simulink model "simmechanics_inverted_pendulum_v6"  (Simulink 7.6)
settings: Solver=ode4  StartTime=0.0  StopTime=10  FixedStep=step_v  RelTol=1e-3
undefined symbols (not defined in the file or in its folder): g
libraries: mblibv1 x21
settings Model: Creator=pierobon  LastModifiedBy=panics
settings DebuggingCC: StrictBusMsg=Warning
settings SimMechanicsCC: VisOnUpdateDiagram=on  VisDuringSimulation=on  AutoFitVis=GROWTOFIT  LastVizWinPosition=[776 162 684 558]  CamPosition=[-14.9891;0.0801796;0.800186;]  CamTarget=[0;0.0801796;0.800186;]  CamUpVector=[0;1;0;]  CamHeight=5.2311  VisBackgroundColor=[0.729412;0.831373;0.956863;]  DefaultBodyColor=[1;0;0;]

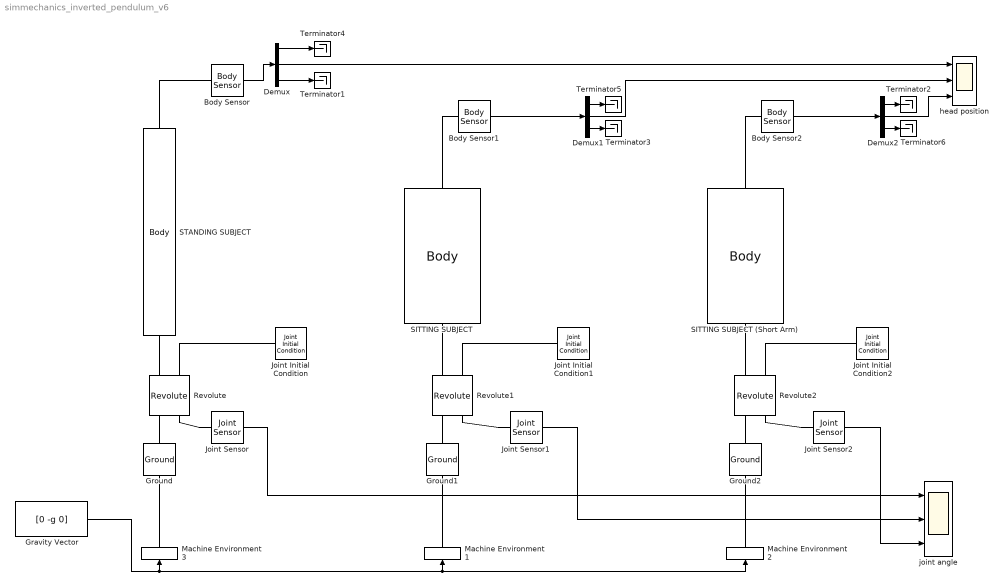
== system simmechanics_inverted_pendulum_v6 ==
  Body Sensor : mblibv1/Sensors &  Actuators/Body Sensor  DialogController=MECH.DynMechDlgSource  SystemSampleTime=-1  UpdateFromCAD=off  PhysicalDomain=Mechanical  PortType=blob  Muxed=off  Pose=off  Angle=on  AngleUnits=deg  ArcVelocity=off  ArcVelocityUnits=deg/s  ArcAcceleration=off  ArcAccelerationUnits=deg/s^2  CoordPosition=on  CoordPositionUnits=in  Velocity=off  VelocityUnits=m/s  Acceleration=off  AccelerationUnits=m/s^2  Quaternion=on  QuaternionDT=off  QuaternionDDT=off  QuaternionUnits=off  OutputVector=[1]  ActiveIO=on  Width=3  DialogClass=MechanicalSensorBlock  ReferenceFrame=Absolute (World)
  Body Sensor1 : mblibv1/Sensors &  Actuators/Body Sensor  DialogController=MECH.DynMechDlgSource  SystemSampleTime=-1  UpdateFromCAD=off  PhysicalDomain=Mechanical  PortType=blob  Muxed=off  Pose=off  Angle=on  AngleUnits=deg  ArcVelocity=off  ArcVelocityUnits=deg/s  ArcAcceleration=off  ArcAccelerationUnits=deg/s^2  CoordPosition=on  CoordPositionUnits=in  Velocity=off  VelocityUnits=m/s  Acceleration=off  AccelerationUnits=m/s^2  Quaternion=on  QuaternionDT=off  QuaternionDDT=off  QuaternionUnits=off  OutputVector=[1]  ActiveIO=on  Width=3  DialogClass=MechanicalSensorBlock  ReferenceFrame=Absolute (World)
  Body Sensor2 : mblibv1/Sensors &  Actuators/Body Sensor  DialogController=MECH.DynMechDlgSource  SystemSampleTime=-1  UpdateFromCAD=off  PhysicalDomain=Mechanical  PortType=blob  Muxed=off  Pose=off  Angle=on  AngleUnits=deg  ArcVelocity=off  ArcVelocityUnits=deg/s  ArcAcceleration=off  ArcAccelerationUnits=deg/s^2  CoordPosition=on  CoordPositionUnits=in  Velocity=off  VelocityUnits=m/s  Acceleration=off  AccelerationUnits=m/s^2  Quaternion=on  QuaternionDT=off  QuaternionDDT=off  QuaternionUnits=off  OutputVector=[1]  ActiveIO=on  Width=3  DialogClass=MechanicalSensorBlock  ReferenceFrame=Absolute (World)
  Demux : Demux  Outputs=3
  Demux1 : Demux  Outputs=3
  Demux2 : Demux  Outputs=3
  Gravity Vector : Constant  Value=[0 -g 0]  VectorParams1D=off
  Ground : mblibv1/Bodies/Ground  DialogController=MECH.DynMechDlgSource  SystemSampleTime=-1  UpdateFromCAD=off  LeftPortType=env  RightPortType=workingframe  PhysicalDomain=Mechanical  DialogClass=GroundBlock  CoordPosition=[0 0 0]  CoordPositionUnits=m  StateVectorMgrId=5  MachineId=[2 2]  ShowEnvPort=on
  Ground1 : mblibv1/Bodies/Ground  DialogController=MECH.DynMechDlgSource  SystemSampleTime=-1  UpdateFromCAD=off  LeftPortType=env  RightPortType=workingframe  PhysicalDomain=Mechanical  DialogClass=GroundBlock  CoordPosition=[0 0 40]  CoordPositionUnits=in  StateVectorMgrId=3  MachineId=[2 0]  ShowEnvPort=on
  Ground2 : mblibv1/Bodies/Ground  DialogController=MECH.DynMechDlgSource  SystemSampleTime=-1  UpdateFromCAD=off  LeftPortType=env  RightPortType=workingframe  PhysicalDomain=Mechanical  DialogClass=GroundBlock  CoordPosition=[0 0 80]  CoordPositionUnits=in  StateVectorMgrId=4  MachineId=[2 1]  ShowEnvPort=on
  Joint Initial Condition : mblibv1/Sensors &  Actuators/Joint Initial Condition  DialogController=MECH.DynMechDlgSource  SystemSampleTime=-1  UpdateFromCAD=off  LeftPortType=blob  RightPortType=blob  PhysicalDomain=mechanical  DialogClass=InitialConditionBlock  InitialConditions=P1$false$0$m$deg$0$m/s$deg/s#P2$false$0$m$deg$0$m/s$deg/s#P3$false$0$m$deg$0$m/s$deg/s#R1$true$IC$m$deg$IV$m/s$deg/s#R2$false$0$m$deg$0$m/s$deg/s#R3$false$0$m$deg$0$m/s$deg/s#S$false$0$m$deg$0$m/s$deg/s  P1PIC=0  P1VIC=0  P2PIC=0  P2VIC=0  P3PIC=0  P3VIC=0  R1PIC=IC  R1VIC=IV  R2PIC=0  R2VIC=0  R3PIC=0  R3VIC=0  SPIC=0  SVIC=0
  Joint Initial Condition1 : mblibv1/Sensors &  Actuators/Joint Initial Condition  DialogController=MECH.DynMechDlgSource  SystemSampleTime=-1  UpdateFromCAD=off  LeftPortType=blob  RightPortType=blob  PhysicalDomain=mechanical  DialogClass=InitialConditionBlock  InitialConditions=P1$false$0$m$deg$0$m/s$deg/s#P2$false$0$m$deg$0$m/s$deg/s#P3$false$0$m$deg$0$m/s$deg/s#R1$true$IC$m$deg$IV$m/s$deg/s#R2$false$0$m$deg$0$m/s$deg/s#R3$false$0$m$deg$0$m/s$deg/s#S$false$0$m$deg$0$m/s$deg/s  P1PIC=0  P1VIC=0  P2PIC=0  P2VIC=0  P3PIC=0  P3VIC=0  R1PIC=IC  R1VIC=IV  R2PIC=0  R2VIC=0  R3PIC=0  R3VIC=0  SPIC=0  SVIC=0
  Joint Initial Condition2 : mblibv1/Sensors &  Actuators/Joint Initial Condition  DialogController=MECH.DynMechDlgSource  SystemSampleTime=-1  UpdateFromCAD=off  LeftPortType=blob  RightPortType=blob  PhysicalDomain=mechanical  DialogClass=InitialConditionBlock  InitialConditions=P1$false$0$m$deg$0$m/s$deg/s#P2$false$0$m$deg$0$m/s$deg/s#P3$false$0$m$deg$0$m/s$deg/s#R1$true$IC$m$deg$IV$m/s$deg/s#R2$false$0$m$deg$0$m/s$deg/s#R3$false$0$m$deg$0$m/s$deg/s#S$false$0$m$deg$0$m/s$deg/s  P1PIC=0  P1VIC=0  P2PIC=0  P2VIC=0  P3PIC=0  P3VIC=0  R1PIC=IC  R1VIC=IV  R2PIC=0  R2VIC=0  R3PIC=0  R3VIC=0  SPIC=0  SVIC=0
  Joint Sensor : mblibv1/Sensors &  Actuators/Joint Sensor  DialogController=MECH.DynMechDlgSource  SystemSampleTime=-1  UpdateFromCAD=off  PhysicalDomain=Mechanical  PortType=blob  Muxed=on  Pose=off  Angle=on  AngleUnits=deg  ArcVelocity=on  ArcVelocityUnits=deg/s  ArcAcceleration=off  ArcAccelerationUnits=deg/s^2  CoordPosition=on  CoordPositionUnits=m  Velocity=off  VelocityUnits=m/s  Acceleration=off  AccelerationUnits=m/s^2  Quaternion=on  QuaternionDT=off  QuaternionDDT=off  QuaternionUnits=off  OutputVector=[1]  ActiveIO=on  Width=2  DialogClass=MechanicalSensorBlock  Primitive=R1  Force=off  ForceUnits=N  Torque=off  TorqueUnits=N*m  ReferenceFrame=Absolute (World)  ReactionSensedSide=Base  ReactionReferenceFrame=Absolute (World)  ReactionForce=off  ReactionForceUnits=N  ReactionMoment=off  ReactionMomentUnits=N*m
  Joint Sensor1 : mblibv1/Sensors &  Actuators/Joint Sensor  DialogController=MECH.DynMechDlgSource  SystemSampleTime=-1  UpdateFromCAD=off  PhysicalDomain=Mechanical  PortType=blob  Muxed=on  Pose=off  Angle=on  AngleUnits=deg  ArcVelocity=on  ArcVelocityUnits=deg/s  ArcAcceleration=off  ArcAccelerationUnits=deg/s^2  CoordPosition=on  CoordPositionUnits=m  Velocity=off  VelocityUnits=m/s  Acceleration=off  AccelerationUnits=m/s^2  Quaternion=on  QuaternionDT=off  QuaternionDDT=off  QuaternionUnits=off  OutputVector=[1]  ActiveIO=on  Width=2  DialogClass=MechanicalSensorBlock  Primitive=R1  Force=off  ForceUnits=N  Torque=off  TorqueUnits=N*m  ReferenceFrame=Absolute (World)  ReactionSensedSide=Base  ReactionReferenceFrame=Absolute (World)  ReactionForce=off  ReactionForceUnits=N  ReactionMoment=off  ReactionMomentUnits=N*m
  Joint Sensor2 : mblibv1/Sensors &  Actuators/Joint Sensor  DialogController=MECH.DynMechDlgSource  SystemSampleTime=-1  UpdateFromCAD=off  PhysicalDomain=Mechanical  PortType=blob  Muxed=on  Pose=off  Angle=on  AngleUnits=deg  ArcVelocity=on  ArcVelocityUnits=deg/s  ArcAcceleration=off  ArcAccelerationUnits=deg/s^2  CoordPosition=on  CoordPositionUnits=m  Velocity=off  VelocityUnits=m/s  Acceleration=off  AccelerationUnits=m/s^2  Quaternion=on  QuaternionDT=off  QuaternionDDT=off  QuaternionUnits=off  OutputVector=[1]  ActiveIO=on  Width=2  DialogClass=MechanicalSensorBlock  Primitive=R1  Force=off  ForceUnits=N  Torque=off  TorqueUnits=N*m  ReferenceFrame=Absolute (World)  ReactionSensedSide=Base  ReactionReferenceFrame=Absolute (World)  ReactionForce=off  ReactionForceUnits=N  ReactionMoment=off  ReactionMomentUnits=N*m
  Machine Environment1 : mblibv1/Bodies/Machine Environment  DialogController=MECH.DialogSource  SystemSampleTime=-1  PortType=env  PhysicalDomain=Mechanical  DialogTemplateClass=MECH.MachineEnvironment  SyncWhenCopied=off  Gravity=[0 g 0 ]  GravityUnits=m/s^2  GravityAsSignal=on  Dimensionality=3D Only  AnalysisType=Forward dynamics  LinearAssemblyTolerance=1e-3  LinearAssemblyToleranceUnits=in  AngularAssemblyTolerance=1e-3  AngularAssemblyToleranceUnits=rad  ConstraintSolverType=Stabilizing  ConstraintRelTolerance=1e-4  ConstraintAbsTolerance=1e-4  UseRobustSingularityHandling=off  RedundancyAnalysisToleranceType=Automatically select tolerance  RedundancyAnalysisTolerance=1e-14  StatePerturbationType=Fixed  PerturbationSize=1e-5  VisualizeMachine=on  BodyVisualizationType=Convex hull from body CS locations  BodyColorSelMode=Use model default  DefaultBodyColor=[1 0 0]
  Machine Environment2 : mblibv1/Bodies/Machine Environment  DialogController=MECH.DialogSource  SystemSampleTime=-1  PortType=env  PhysicalDomain=Mechanical  DialogTemplateClass=MECH.MachineEnvironment  SyncWhenCopied=off  Gravity=[0 g 0 ]  GravityUnits=m/s^2  GravityAsSignal=on  Dimensionality=3D Only  AnalysisType=Forward dynamics  LinearAssemblyTolerance=1e-3  LinearAssemblyToleranceUnits=in  AngularAssemblyTolerance=1e-3  AngularAssemblyToleranceUnits=rad  ConstraintSolverType=Stabilizing  ConstraintRelTolerance=1e-4  ConstraintAbsTolerance=1e-4  UseRobustSingularityHandling=off  RedundancyAnalysisToleranceType=Automatically select tolerance  RedundancyAnalysisTolerance=1e-14  StatePerturbationType=Fixed  PerturbationSize=1e-5  VisualizeMachine=on  BodyVisualizationType=Convex hull from body CS locations  BodyColorSelMode=Use model default  DefaultBodyColor=[1 0 0]
  Machine Environment3 : mblibv1/Bodies/Machine Environment  DialogController=MECH.DialogSource  SystemSampleTime=-1  PortType=env  PhysicalDomain=Mechanical  DialogTemplateClass=MECH.MachineEnvironment  SyncWhenCopied=off  Gravity=[0 g 0 ]  GravityUnits=m/s^2  GravityAsSignal=on  Dimensionality=3D Only  AnalysisType=Forward dynamics  LinearAssemblyTolerance=1e-3  LinearAssemblyToleranceUnits=in  AngularAssemblyTolerance=1e-3  AngularAssemblyToleranceUnits=rad  ConstraintSolverType=Stabilizing  ConstraintRelTolerance=1e-4  ConstraintAbsTolerance=1e-4  UseRobustSingularityHandling=off  RedundancyAnalysisToleranceType=Automatically select tolerance  RedundancyAnalysisTolerance=1e-14  StatePerturbationType=Fixed  PerturbationSize=1e-5  VisualizeMachine=on  BodyVisualizationType=Convex hull from body CS locations  BodyColorSelMode=Use model default  DefaultBodyColor=[1 0 0]
  Revolute : mblibv1/Joints/Revolute  DialogController=MECH.DynMechDlgSource  PhysicalDomain=mechanical  SubClassName=Unknown  LeftPortType=blob  RightPortType=blob  LConnTagsString=__newl0|SA1  RConnTagsString=__newr0|SA1  UpdateFromCAD=off  NumSAPorts=2  CutJoint=off  MarkAsCut=off  Primitives=prismatic  PrimitiveProps=R1$World$[1 0 0]$revolute  DialogClass=JointBlock  R1Axis=[1 0 0]
  Revolute1 : mblibv1/Joints/Revolute  DialogController=MECH.DynMechDlgSource  PhysicalDomain=mechanical  SubClassName=Unknown  LeftPortType=blob  RightPortType=blob  LConnTagsString=__newl0|SA1  RConnTagsString=__newr0|SA1  UpdateFromCAD=off  NumSAPorts=2  CutJoint=off  MarkAsCut=off  Primitives=prismatic  PrimitiveProps=R1$World$[1 0 0]$revolute  DialogClass=JointBlock  R1Axis=[1 0 0]
  Revolute2 : mblibv1/Joints/Revolute  DialogController=MECH.DynMechDlgSource  PhysicalDomain=mechanical  SubClassName=Unknown  LeftPortType=blob  RightPortType=blob  LConnTagsString=__newl0|SA1  RConnTagsString=__newr0|SA1  UpdateFromCAD=off  NumSAPorts=2  CutJoint=off  MarkAsCut=off  Primitives=prismatic  PrimitiveProps=R1$World$[1 0 0]$revolute  DialogClass=JointBlock  R1Axis=[1 0 0]
  SITTING SUBJECT : mblibv1/Bodies/Body  DialogController=MECH.DynMechDlgSource  PhysicalDomain=mechanical  SubClassName=Unknown  LeftPortType=workingframe  RightPortType=workingframe  LConnTagsString=CS1  RConnTagsString=CS2  UpdateFromCAD=off  DialogClass=MechanicalBodyBlock  Mass=166.4  MassUnits=lbm  InertiaUnits=lbm*in^2  Inertia=[61.1 0 0; 0 33.5 0; 0 0 66.6]  Shape=Cylinder  ShapeDims=[1 1]  ShapeUnits=m  ShapeUse=false  Density=1  DensityUnits=kg/m^3  DensityUse=false  GraphicsMode=CONVHULL  BodyColorSelMode=COLORPALETTE  BodyColor=[1 0 0]  AttachedToCS=CG  CG=Left$CG$[0 21.4 0]$CS1$CS1$in$[0 0 0]$Euler X-Y-Z$deg$WORLD$false$none  WorkingFrames="Left$CS1$[0 0 40]$World$World$in$[0 0 0]$Euler X-Y-Z$deg$WORLD$true$none#Right$CS2$[0  26.5 0]$CG$CG$in$[0 0 0]$Euler X-Y-Z$deg$WORLD$true$none#Left$CS3$[0 0 -7.9]$CG$CG$in$[0 0 0]$Euler X-Y-Z$deg$WORLD$false$none#Left$CS4$[0 26.5 -7.9]$CG$CG$in$[0 0 0]$Euler X-Y-Z$deg$WORLD$false$none#Left$CS5$[0 26.5 3.5]$CG$CG$in$[0 0 0]$Euler X-Y-Z$deg$WORLD$false$none#Left$CS6$[0 0 21.4]$CG$CG$in$[0 0 0]$Euler X-Y-Z$deg$WORLD$false$none#Left$CS7$[0 0 21.4]$CS1$CS1$in$[0 0 0]$Euler X-Y-Z$deg$WORLD$false$none"  CGPos=[0 21.4 0]  CGRot=[0 0 0]  CS0Pos=[]  CS0Rot=[]  CS1Pos=[0 0 40]  CS1Rot=[0 0 0]  CS2Pos="[0  26.5 0]"  CS2Rot=[0 0 0]  CS3Pos=[0 0 -7.9]  CS3Rot=[0 0 0]  CS4Pos=[0 26.5 -7.9]  CS4Rot=[0 0 0]  CS5Pos=[0 26.5 3.5]  CS5Rot=[0 0 0]  CS6Pos=[0 0 21.4]  CS6Rot=[0 0 0]  CS7Pos=[0 0 21.4]  CS7Rot=[0 0 0]  CS8Pos=[]  CS8Rot=[]  CS9Pos=[]  CS9Rot=[]  CS10Pos=[]  CS10Rot=[]  CS11Pos=[]  CS11Rot=[]  CS12Pos=[]  CS12Rot=[]  CS13Pos=[]  CS13Rot=[]  CS14Pos=[]  CS14Rot=[]  CS15Pos=[]  CS15Rot=[]  CS16Pos=[]  CS16Rot=[]  CS17Pos=[]  CS17Rot=[]  CS18Pos=[]  CS18Rot=[]  CS19Pos=[]  CS19Rot=[]  CS20Pos=[]  CS20Rot=[]
  SITTING SUBJECT (Short Arm) : mblibv1/Bodies/Body  DialogController=MECH.DynMechDlgSource  PhysicalDomain=mechanical  SubClassName=Unknown  LeftPortType=workingframe  RightPortType=workingframe  LConnTagsString=CS1  RConnTagsString=CS2  UpdateFromCAD=off  DialogClass=MechanicalBodyBlock  Mass=166.4  MassUnits=lbm  InertiaUnits=lbm*in^2  Inertia=[61.1 0 0; 0 33.5 0; 0 0 66.6]  Shape=Cylinder  ShapeDims=[1 1]  ShapeUnits=m  ShapeUse=false  Density=1  DensityUnits=kg/m^3  DensityUse=false  GraphicsMode=CONVHULL  BodyColorSelMode=COLORPALETTE  BodyColor=[0 0.74902 0.74902]  AttachedToCS=CG  CG=Left$CG$[0 3.5 0]$CS1$CS1$in$[0 0 0]$Euler X-Y-Z$deg$WORLD$false$none  WorkingFrames="Left$CS1$[0 0 80]$World$World$in$[0 0 0]$Euler X-Y-Z$deg$WORLD$true$none#Right$CS2$[0  26.5 0]$CG$CG$in$[0 0 0]$Euler X-Y-Z$deg$WORLD$true$none#Left$CS3$[0 0 -7.9]$CG$CG$in$[0 0 0]$Euler X-Y-Z$deg$WORLD$false$none#Left$CS4$[0 26.5 -7.9]$CG$CG$in$[0 0 0]$Euler X-Y-Z$deg$WORLD$false$none#Left$CS5$[0 26.5 3.5]$CG$CG$in$[0 0 0]$Euler X-Y-Z$deg$WORLD$false$none#Left$CS6$[0 0 21.4]$CG$CG$in$[0 0 0]$Euler X-Y-Z$deg$WORLD$false$none#Left$CS7$[0 -21.4 21.4]$CG$CG$in$[0 0 0]$Euler X-Y-Z$deg$WORLD$false$none#Left$CS8$[0 -21.4 0]$CG$CG$in$[0 0 0]$Euler X-Y-Z$deg$WORLD$false$none"  CGPos=[0 3.5 0]  CGRot=[0 0 0]  CS0Pos=[]  CS0Rot=[]  CS1Pos=[0 0 80]  CS1Rot=[0 0 0]  CS2Pos="[0  26.5 0]"  CS2Rot=[0 0 0]  CS3Pos=[0 0 -7.9]  CS3Rot=[0 0 0]  CS4Pos=[0 26.5 -7.9]  CS4Rot=[0 0 0]  CS5Pos=[0 26.5 3.5]  CS5Rot=[0 0 0]  CS6Pos=[0 0 21.4]  CS6Rot=[0 0 0]  CS7Pos=[0 -21.4 21.4]  CS7Rot=[0 0 0]  CS8Pos=[0 -21.4 0]  CS8Rot=[0 0 0]  CS9Pos=[]  CS9Rot=[]  CS10Pos=[]  CS10Rot=[]  CS11Pos=[]  CS11Rot=[]  CS12Pos=[]  CS12Rot=[]  CS13Pos=[]  CS13Rot=[]  CS14Pos=[]  CS14Rot=[]  CS15Pos=[]  CS15Rot=[]  CS16Pos=[]  CS16Rot=[]  CS17Pos=[]  CS17Rot=[]  CS18Pos=[]  CS18Rot=[]  CS19Pos=[]  CS19Rot=[]  CS20Pos=[]  CS20Rot=[]
  STANDING SUBJECT : mblibv1/Bodies/Body  DialogController=MECH.DynMechDlgSource  PhysicalDomain=mechanical  SubClassName=Unknown  LeftPortType=workingframe  RightPortType=workingframe  LConnTagsString=CS1  RConnTagsString=CS5  UpdateFromCAD=off  DialogClass=MechanicalBodyBlock  Mass=166.4  MassUnits=lbm  InertiaUnits=lbm*in^2  Inertia=[115 0 0; 0 11.3 0; 0 0 103]  Shape=Cylinder  ShapeDims=[1 1]  ShapeUnits=m  ShapeUse=false  Density=1  DensityUnits=kg/m^3  DensityUse=false  GraphicsMode=CONVHULL  BodyColorSelMode=COLORPALETTE  BodyColor="[0     0.49804           0]"  AttachedToCS=CG  CG=Left$CG$[0 38.4 0]$CS1$CS1$in$[0 0 0]$Euler X-Y-Z$deg$WORLD$false$none  WorkingFrames="Left$CS1$[0 0 0]$World$World$in$[0 0 0]$Euler X-Y-Z$deg$WORLD$true$none#Right$CS2$[0  0 -2]$CS1$CS1$in$[0 0 0]$Euler X-Y-Z$deg$WORLD$false$none#Right$CS3$[0  38.4 -3.5]$CS1$CS1$in$[0 0 0]$Euler X-Y-Z$deg$WORLD$false$none#Right$CS4$[0  69.4 -2]$CS1$CS1$in$[0 0 0]$Euler X-Y-Z$deg$WORLD$false$none#Right$CS5$[0  69.4 0]$CS1$CS1$in$[0 0 0]$Euler X-Y-Z$deg$WORLD$true$none#Right$CS6$[0  69.4 2]$CS1$CS1$in$[0 0 0]$Euler X-Y-Z$deg$WORLD$false$none#Right$CS7$[0  38.4 3.5]$CS1$CS1$in$[0 0 0]$Euler X-Y-Z$deg$WORLD$false$none#Right$CS8$[0  0 2]$CS1$CS1$in$[0 0 0]$Euler X-Y-Z$deg$WORLD$false$none"  CGPos=[0 38.4 0]  CGRot=[0 0 0]  CS0Pos=[]  CS0Rot=[]  CS1Pos=[0 0 0]  CS1Rot=[0 0 0]  CS2Pos="[0  0 -2]"  CS2Rot=[0 0 0]  CS3Pos="[0  38.4 -3.5]"  CS3Rot=[0 0 0]  CS4Pos="[0  69.4 -2]"  CS4Rot=[0 0 0]  CS5Pos="[0  69.4 0]"  CS5Rot=[0 0 0]  CS6Pos="[0  69.4 2]"  CS6Rot=[0 0 0]  CS7Pos="[0  38.4 3.5]"  CS7Rot=[0 0 0]  CS8Pos="[0  0 2]"  CS8Rot=[0 0 0]  CS9Pos=[]  CS9Rot=[]  CS10Pos=[]  CS10Rot=[]  CS11Pos=[]  CS11Rot=[]  CS12Pos=[]  CS12Rot=[]  CS13Pos=[]  CS13Rot=[]  CS14Pos=[]  CS14Rot=[]  CS15Pos=[]  CS15Rot=[]  CS16Pos=[]  CS16Rot=[]  CS17Pos=[]  CS17Rot=[]  CS18Pos=[]  CS18Rot=[]  CS19Pos=[]  CS19Rot=[]  CS20Pos=[]  CS20Rot=[]
  Terminator{1..6} (6 alike) : Terminator
  head position : Scope  NumInputPorts=3
      settings: TimeRange=1.5  YMin=-100~-100~-100  YMax=100~100~100
  joint angle : Scope  NumInputPorts=3
      settings: TimeRange=1.5  YMin=-200~-200~-1000  YMax=400~500~1000  SaveName=Joint_angle
  wires:
  Body Sensor/1 -> Demux/1
  Joint Sensor/1 -> joint angle/1
  Body Sensor1/1 -> Demux1/1
  Joint Sensor1/1 -> joint angle/2
  Demux/1 -> Terminator4/1
  Demux/2 -> head position/1
  Demux/3 -> Terminator1/1
  Demux1/2 -> head position/2
  Demux1/3 -> Terminator3/1
  Demux1/1 -> Terminator5/1
  Body Sensor2/1 -> Demux2/1
  Joint Sensor2/1 -> joint angle/3
  Demux2/2 -> head position/3
  Demux2/3 -> Terminator6/1
  Demux2/1 -> Terminator2/1
  Gravity Vector/1 -> Machine Environment3/1, Machine Environment1/1, Machine Environment2/1
  connections:
  Revolute/RConn1 -- STANDING SUBJECT/LConn1
  Ground/RConn1 -- Revolute/LConn1
  Joint Sensor/LConn1 -- Revolute/LConn2
  Joint Initial Condition/RConn1 -- Revolute/RConn2
  Revolute1/RConn1 -- SITTING SUBJECT/LConn1
  Body Sensor1/LConn1 -- SITTING SUBJECT/RConn1
  Ground1/RConn1 -- Revolute1/LConn1
  Joint Initial Condition1/RConn1 -- Revolute1/RConn2
  Joint Sensor1/LConn1 -- Revolute1/LConn2
  Body Sensor/LConn1 -- STANDING SUBJECT/RConn1
  Ground2/RConn1 -- Revolute2/LConn1
  Revolute2/RConn1 -- SITTING SUBJECT (Short Arm)/LConn1
  Body Sensor2/LConn1 -- SITTING SUBJECT (Short Arm)/RConn1
  Joint Sensor2/LConn1 -- Revolute2/LConn2
  Joint Initial Condition2/RConn1 -- Revolute2/RConn2
  Machine Environment3/RConn1 -- Ground/LConn1
  Machine Environment1/RConn1 -- Ground1/LConn1
  Machine Environment2/RConn1 -- Ground2/LConn1
